simulink model "Motor_1"  (R2015a)
settings: Solver=ode45  StartTime=0.0  StopTime=10.0  RelTol=1e-3
settings Model: Creator=Henry Alberto  LastModifiedBy=Henry Alberto

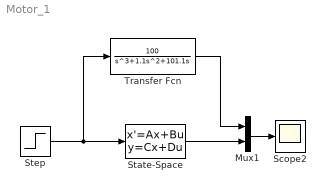
== system Motor_1 ==
  Mux1 : Mux  Inputs=2
  Scope2 : Scope
      settings: SaveName=ScopeData2
  State-Space : StateSpace  A=[0 1 0;0 0 1;0 -101.1 -1.1]  B=[0;0;100]  C=[1 0 0]  D=[0]  X0=0
  Step : Step  SampleTime=0
  Transfer Fcn : TransferFcn  Numerator=[100]  Denominator=[1 1.1 101.1 0]
  wires:
  Transfer Fcn/1 -> Mux1/1
  Step/1 -> Transfer Fcn/1, State-Space/1
  Mux1/1 -> Scope2/1
  State-Space/1 -> Mux1/2
